simulink model "problem1G"  (R2023a)
settings: Solver=VariableStepAuto  StartTime=0.0  StopTime=8  RelTol=1e-3
settings Model: Creator=jadenmecham  LastModifiedBy=jadenmecham

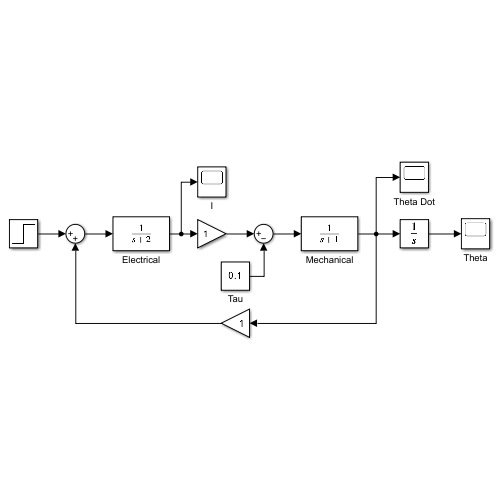
[thumbnail: Simulink's stored preview of the top-level diagram]
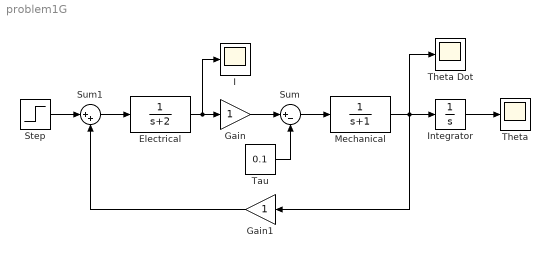
== system problem1G ==
  Electrical : TransferFcn  Denominator=[1 2]
  Gain : Gain
  Gain1 : Gain
  I : Scope
  Integrator : Integrator
  Mechanical : TransferFcn  Denominator=[1 1]
  Step : Step  SampleTime=0
  Sum : Sum  Inputs=|+-
  Sum1 : Sum  Inputs=|++
  Tau : Constant  Value=0.1
  Theta : Scope
  Theta Dot : Scope
  wires:
  Electrical/1 -> I/1, Gain/1
  Gain/1 -> Sum/1
  Tau/1 -> Sum/2
  Sum/1 -> Mechanical/1
  Mechanical/1 -> Theta Dot/1, Gain1/1, Integrator/1
  Integrator/1 -> Theta/1
  Gain1/1 -> Sum1/2
  Step/1 -> Sum1/1
  Sum1/1 -> Electrical/1
